simulink model "on_off_lampara"  (R2018a)
settings: Solver=VariableStepAuto  StartTime=0.0  StopTime=inf  RelTol=1e-3
settings Model: Creator=carma  LastModifiedBy=carma

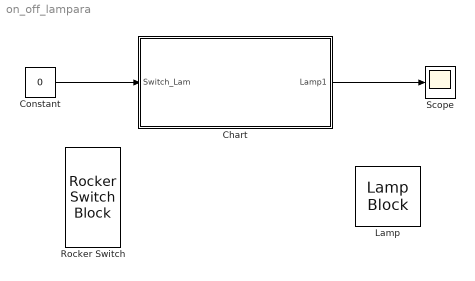
== system on_off_lampara ==
  Chart : Stateflow chart  TreatAsAtomicUnit=on
  Constant : Constant  Value=0
  Lamp : LampBlock  WebBlockId=5
  Rocker Switch : RockerSwitchBlock  WebBlockId=4
      settings: Values={{'Off', 'On'}, [0 1]}
  Scope : Scope
  wires:
  Constant/1 -> Chart/1(Switch_Lam)
  Chart/1(Lamp1) -> Scope/1

== stateflow chart on_off_lampara/Chart ==
  state ON
    entry:
    Lamp1=1;
  state OFF
    entry:
    Lamp1=0;
  (default) -> OFF
  ON -> OFF : [Switch_Lam==0]
  OFF -> ON : [Switch_Lam==1]
  data: Switch_Lam input; Lamp1 output
